simulink model "Reset_test"  (R2023b)
settings: Solver=VariableStepAuto  StartTime=0.0  StopTime=10.0  RelTol=1e-3
undefined symbols (not defined in the file or in its folder): DiscIntNeverNeededParam
settings Model: Creator=diego  LastModifiedBy=diego

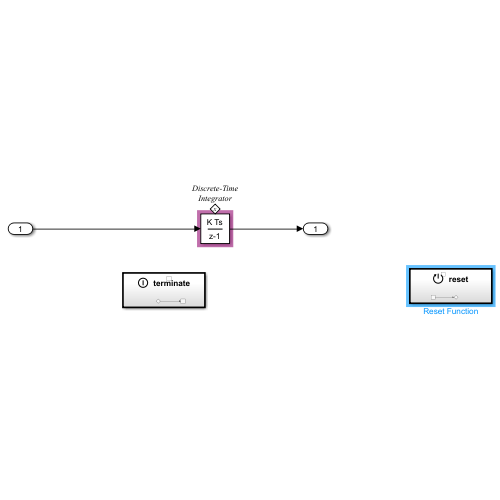
[thumbnail: Simulink's stored preview of the top-level diagram]
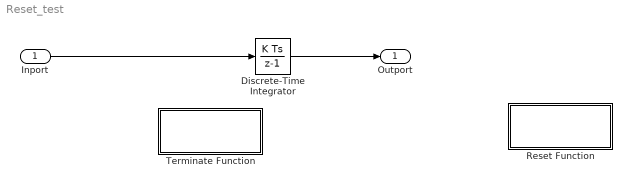
== system Reset_test ==
  Inport : Inport
  Discrete-Time Integrator : DiscreteIntegrator  SampleTime=-1  ICPrevOutput=DiscIntNeverNeededParam  ICPrevScaledInput=DiscIntNeverNeededParam
  Reset Function : Subsystem  TreatAsAtomicUnit=on
  Terminate Function : Subsystem  TreatAsAtomicUnit=on
  Outport : Outport
  wires:
  Inport/1 -> Discrete-Time Integrator/1
  Discrete-Time Integrator/1 -> Outport/1

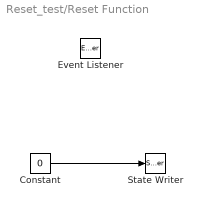
== system Reset_test/Reset Function ==
  Constant : Constant  Value=0
  Event Listener : EventListener  DisableCoverage=on  EventType=Reinitialize  EventName=reset
  State Writer : StateWriter  StateOwnerBlock=../../Discrete-Time Integrator
  wires:
  Constant/1 -> State Writer/1

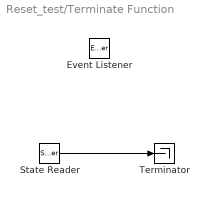
== system Reset_test/Terminate Function ==
  Event Listener : EventListener  DisableCoverage=on  EventType=Terminate  EventName=reset
  State Reader : StateReader  StateOwnerBlock=../../Discrete-Time Integrator
  Terminator : Terminator
  wires:
  State Reader/1 -> Terminator/1
